simulink model "RegulationWithSaturatedInputExample"  (R2018a)
settings: Solver=VariableStepAuto  StartTime=0.0  StopTime=5  RelTol=1e-3
settings Model: Creator=efrem  LastModifiedBy=efrem

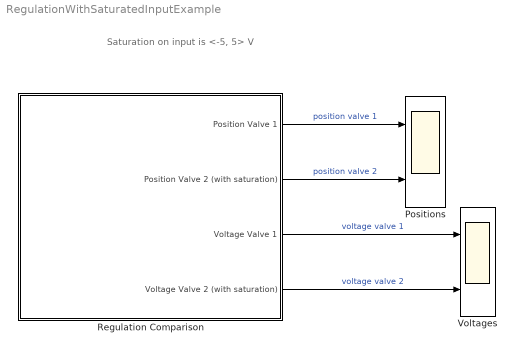
== system RegulationWithSaturatedInputExample ==
  note: Saturation on input is <-5, 5> V
  Positions : Scope  NumInputPorts=2
  Regulation Comparison : Subsystem  mask{k=1.100}
      mask prompts: k "P gain"
  Voltages : Scope  NumInputPorts=2
  wires:
  Regulation Comparison/1(Position Valve 1) -> Positions/1  "position valve 1"
  Regulation Comparison/2(Position Valve 2 (with saturation)) -> Positions/2  "position valve 2"
  Regulation Comparison/3(Voltage Valve 1) -> Voltages/1  "voltage valve 1"
  Regulation Comparison/4(Voltage Valve 2 (with saturation)) -> Voltages/2  "voltage valve 2"

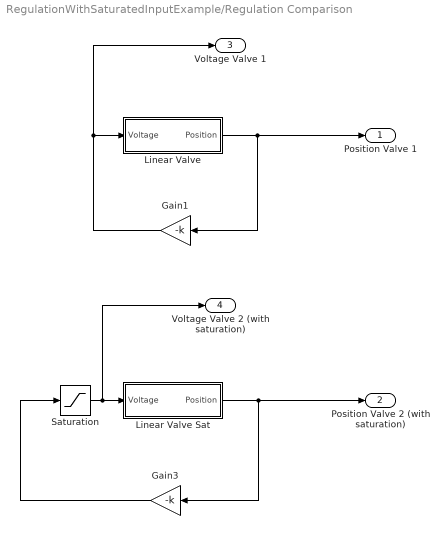
== system RegulationWithSaturatedInputExample/Regulation Comparison ==
  Gain1 : Gain  Gain=-k
  Gain3 : Gain  Gain=-k
  Linear Valve : Subsystem
  Linear Valve Sat : Subsystem
  Saturation : Saturate  UpperLimit=5  LowerLimit=-5
  Position Valve 1 : Outport
  Position Valve 2 (with saturation) : Outport  Port=2
  Voltage Valve 1 : Outport  Port=3
  Voltage Valve 2 (with saturation) : Outport  Port=4
  wires:
  Linear Valve Sat/1(Position) -> Position Valve 2 (with saturation)/1, Gain3/1
  Saturation/1 -> Voltage Valve 2 (with saturation)/1, Linear Valve Sat/1(Voltage)
  Gain3/1 -> Saturation/1
  Gain1/1 -> Voltage Valve 1/1, Linear Valve/1(Voltage)
  Linear Valve/1(Position) -> Position Valve 1/1, Gain1/1

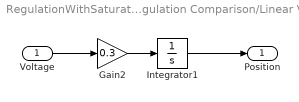
== system RegulationWithSaturatedInputExample/Regulation Comparison/Linear Valve ==
  Voltage : Inport
  Gain2 : Gain  Gain=0.3
  Integrator1 : Integrator  InitialCondition=1  LimitOutput=on  UpperSaturationLimit=1  LowerSaturationLimit=0
  Position : Outport
  wires:
  Gain2/1 -> Integrator1/1
  Voltage/1 -> Gain2/1
  Integrator1/1 -> Position/1

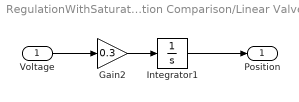
== system RegulationWithSaturatedInputExample/Regulation Comparison/Linear Valve Sat ==
  Voltage : Inport
  Gain2 : Gain  Gain=0.3
  Integrator1 : Integrator  InitialCondition=1  LimitOutput=on  UpperSaturationLimit=1  LowerSaturationLimit=0
  Position : Outport
  wires:
  Gain2/1 -> Integrator1/1
  Voltage/1 -> Gain2/1
  Integrator1/1 -> Position/1
